simulink model "SimpleTank"  (Simulink 7.6)
settings: Solver=ode45  StartTime=0.0  StopTime=10000000000.0  RelTol=1e-3
values from neighbouring files (symbols this model uses):
  coldflow = 20    [init.m]
  constants = [T_cold, T_hot, alpha]    [init.m]
undefined symbols (not defined in the file or in its folder): Newton, Raphson
settings Model: Creator=oliverst  LastModifiedBy=ost

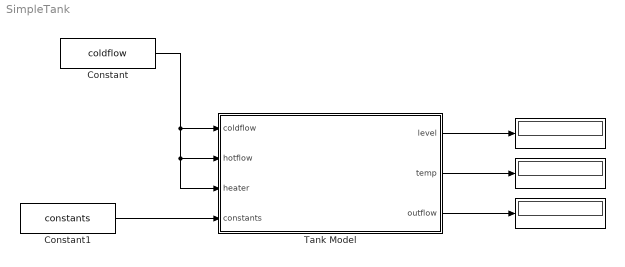
== system SimpleTank ==
  "                                        " : Display
  "                                           " : Display
  "                                               " : Display
  Constant : Constant  Value=coldflow
  Constant1 : Constant  Value=constants
  Tank Model : Subsystem
  wires:
  Tank Model/1(level) -> "                                        "/1
  Tank Model/2(temp) -> "                                           "/1
  Tank Model/3(outflow) -> "                                               "/1
  Constant/1 -> Tank Model/1(coldflow), Tank Model/2(hotflow), Tank Model/3(heater)
  Constant1/1 -> Tank Model/4(constants)

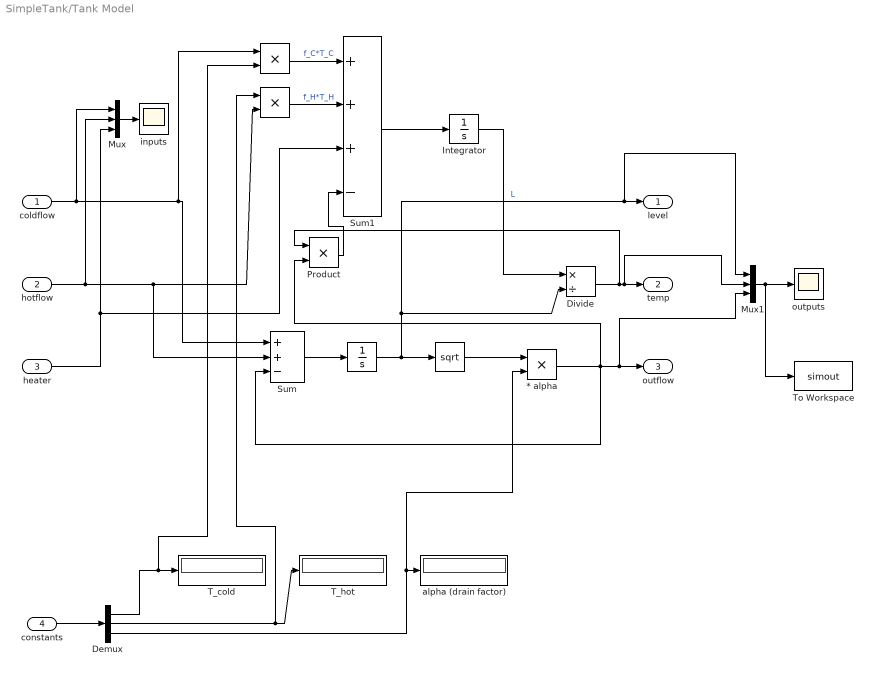
== system SimpleTank/Tank Model ==
  coldflow : Inport
  hotflow : Inport  Port=2
  heater : Inport  Port=3
  constants : Inport  Port=4
  " " : Sqrt  AlgorithmType=Newton-Raphson  SaturateOnIntegerOverflow=on
  "   " : Integrator  InitialCondition=1
  "     " : Product  RndMeth=Zero
  "               " : Product  RndMeth=Zero
  * alpha : Product  RndMeth=Zero
  Demux : Demux  Outputs=3
  Divide : Product  Inputs=*/
  Integrator : Integrator  InitialCondition=1
  Mux : Mux  Inputs=3
  Mux1 : Mux  Inputs=3
  Product : Product  RndMeth=Zero
  Sum : Sum  Inputs=++-
  Sum1 : Sum  Inputs=+++-
  T_cold : Display
  T_hot : Display
  To Workspace : ToWorkspace  VariableName=simout  SampleTime=-1  SaveFormat=Structure
  alpha (drain factor) : Display
  inputs : Scope
      settings: TimeRange=10000  YMin=20  YMax=20
  outputs : Scope
      settings: TimeRange=10000  YMin=0  YMax=2500
  level : Outport
  temp : Outport  Port=2
  outflow : Outport  Port=3
  wires:
  constants/1 -> Demux/1
  Demux/1 -> T_cold/1, "               "/2
  Demux/2 -> T_hot/1, "     "/1
  Mux/1 -> inputs/1
  coldflow/1 -> Mux/1, Sum/1, "               "/1
  hotflow/1 -> Mux/2, Sum/2, "     "/2
  heater/1 -> Mux/3, Sum1/3
  Demux/3 -> alpha (drain factor)/1, * alpha/2
  " "/1 -> * alpha/1
  "   "/1 -> " "/1, Divide/2, level/1, Mux1/1  "L"
  * alpha/1 -> Sum/3, Product/2, outflow/1, Mux1/3
  Sum/1 -> "   "/1
  "     "/1 -> Sum1/2  "f_H*T_H"
  "               "/1 -> Sum1/1  "f_C*T_C"
  Product/1 -> Sum1/4
  Divide/1 -> Product/1, temp/1, Mux1/2
  Sum1/1 -> Integrator/1
  Integrator/1 -> Divide/1
  Mux1/1 -> outputs/1, To Workspace/1
